simulink model "kaskada"  (R2020b)
settings: Solver=ode45  StartTime=0.0  StopTime=10.0  RelTol=1e-3  EnableMultiTasking=on
undefined symbols (not defined in the file): B, In, J, Kp, KT, Kw, m, psie, psie1, R, R1, T, Un, V, Y
settings Model: Creator=Konrad  LastModifiedBy=Dom
settings DataIOCC: LimitDataPoints=on  SaveFormat=Array  SignalLoggingSaveFormat=ModelDataLogs  ReturnWorkspaceOutputs=off
settings OptimizationCC: ExpressionDepthLimit=2147483647  LifeSpan=inf
settings DebuggingCC: UnderspecifiedInitializationDetection=Classic  MergeDetectMultiDrivingBlocksExec=none  SolverPrmCheckMsg=warning  FcnCallInpInsideContextMsg=warning  StateNameClashWarn=warning  SFUnexpectedBacktrackingDiag=warning  SFNoUnconditionalDefaultTransitionDiag=warning  ArithmeticOperatorsInVariantConditions=warning
settings HardwareCC: ProdBitPerPointer=32  ProdBitPerSizeT=32  ProdBitPerPtrDiffT=32  ProdLargestAtomicFloat=None  ProdIntDivRoundTo=Undefined  ProdEndianess=Unspecified  ProdWordSize=32  ProdHWDeviceType=32-bit Generic
settings ModelReferenceCC: PropagateSignalLabelsOutOfModel=off
settings SFSimCC: SimUseLocalCustomCode=off  CustomCodeUndefinedFunction=UseInterfaceOnly
settings RTWCC: RTWUseLocalCustomCode=off
settings CodeAppCC: StateflowObjectComments=on
settings GRTTargetCC: TargetLangStandard=C89/C90 (ANSI)  CombineOutputUpdateFcns=off  GRTInterface=on
settings ConfigComp: CovMetricSettings=dw  CovSaveCumulativeToWorkspaceVar=on  CovSaveSingleToWorkspaceVar=on  CovExternalEMLEnable=off

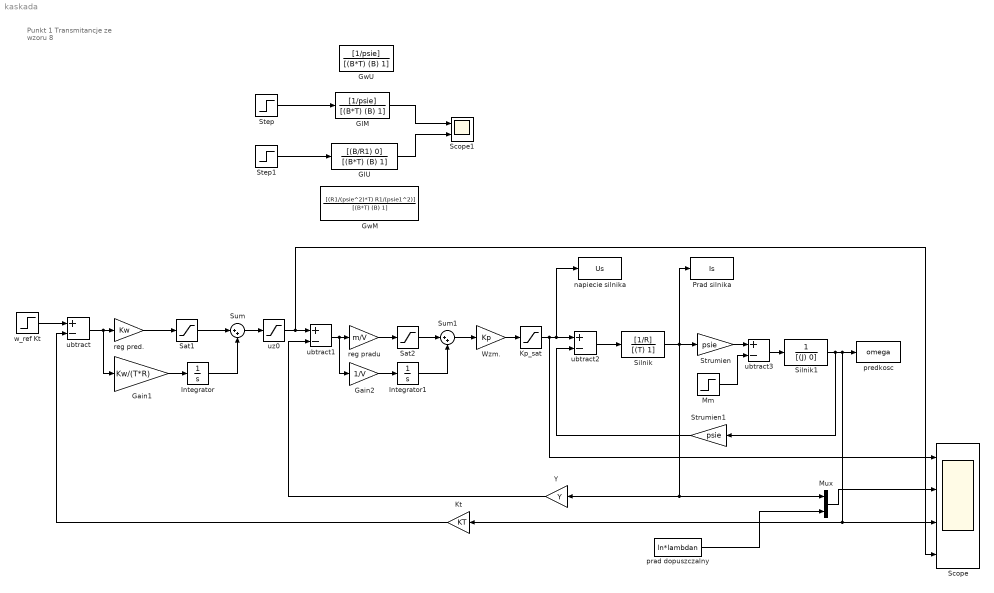
== system kaskada ==
  note: Punkt 1
      | Transmitancje ze wzoru 8
  GIM : TransferFcn  Numerator=[1/psie]  Denominator=[(B*T) (B) 1]
  GIU : TransferFcn  Numerator=[(B/R1) 0]  Denominator=[(B*T) (B) 1]
  Gain1 : Gain  Gain=Kw/(T*R)
  Gain2 : Gain  Gain=1/V
  GwM : TransferFcn  Numerator=[(R1/(psie^2)*T) R1/(psie1^2)]  Denominator=[(B*T) (B) 1]
  GwU : TransferFcn  Numerator=[1/psie]  Denominator=[(B*T) (B) 1]
  Integrator : Integrator  LimitOutput=on  UpperSaturationLimit=1  LowerSaturationLimit=0
  Integrator1 : Integrator  LimitOutput=on  UpperSaturationLimit=1  LowerSaturationLimit=0
  Kp_sat : Saturate
  Kt : Gain  Gain=KT
  Mm : Step  SampleTime=0
  Mux : Mux  Inputs=2
  Prad silnika : ToWorkspace  VariableName=Is  SaveFormat=Structure  SampleTime=-1
  Sat1 : Saturate  UpperLimit=10  LowerLimit=-10
  Sat2 : Saturate  UpperLimit=10  LowerLimit=-10
  Scope : Scope  NumInputPorts=4
  Scope1 : Scope  NumInputPorts=2
  Silnik : TransferFcn  Numerator=[1/R]  Denominator=[(T) 1]
  Silnik1 : TransferFcn  Denominator=[(J) 0]
  Step : Step  After=2*In  SampleTime=0
  Step1 : Step  After=Un  SampleTime=0
  Strumien : Gain  Gain=psie
  Strumien1 : Gain  Gain=psie
  Sum : Sum  Inputs=|++
  Sum1 : Sum  Inputs=|++
  Wzm. : Gain  Gain=Kp
  Y : Gain  Gain=Y
  napiecie silnika : ToWorkspace  VariableName=Us  SaveFormat=Structure  SampleTime=-1
  prad dopuszczalny : FromWorkspace  VariableName=ln*lambdan
  predkosc : ToWorkspace  VariableName=omega  SaveFormat=Structure  SampleTime=-1
  reg pradu : Gain  Gain=m/V
  reg pred. : Gain  Gain=Kw
  ubtract{,1..3} (4 alike) : Sum  Inputs=+-
  uz0 : Saturate  UpperLimit=5  LowerLimit=-5
  w_ref Kt : Step  After=Un  SampleTime=0
  wires:
  w_ref Kt/1 -> ubtract/1
  ubtract/1 -> reg pred./1, Gain1/1
  reg pred./1 -> Sat1/1
  Sat1/1 -> Sum/1
  Gain1/1 -> Integrator/1
  Integrator/1 -> Sum/2
  Sum/1 -> uz0/1
  uz0/1 -> ubtract1/1, Scope/4
  ubtract1/1 -> reg pradu/1, Gain2/1
  reg pradu/1 -> Sat2/1
  Sat2/1 -> Sum1/1
  Gain2/1 -> Integrator1/1
  Integrator1/1 -> Sum1/2
  Sum1/1 -> Wzm./1
  Wzm./1 -> Kp_sat/1
  Kp_sat/1 -> ubtract2/1, napiecie silnika/1, Scope/1
  ubtract2/1 -> Silnik/1
  Silnik/1 -> Strumien/1, Prad silnika/1, Mux/1, Y/1
  Strumien/1 -> ubtract3/1
  Mm/1 -> ubtract3/2
  ubtract3/1 -> Silnik1/1
  Silnik1/1 -> predkosc/1, Scope/3, Kt/1, Strumien1/1
  Mux/1 -> Scope/2
  prad dopuszczalny/1 -> Mux/2
  Strumien1/1 -> ubtract2/2
  Y/1 -> ubtract1/2
  Kt/1 -> ubtract/2
  GIM/1 -> Scope1/1
  GIU/1 -> Scope1/2
  Step1/1 -> GIU/1
  Step/1 -> GIM/1
